simulink model "piddiscreto"  (Simulink 4.00)
settings: Solver=ode45  StartTime=0.0  StopTime=10.0  RelTol=1e-3
settings Model: LastModifiedBy=Gui

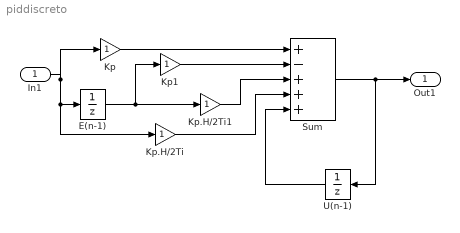
== system piddiscreto ==
  In1 : Inport  Port=1  LatchInput=off
  E(n-1) : UnitDelay  X0=0  SampleTime=0.005
      settings: RTWStateStorageClass=Auto
  Kp : Gain  Gain=1  Multiplication=Element-wise(K.*u)  SaturateOnIntegerOverflow=on
  Kp.H/2Ti : Gain  Gain=1  Multiplication=Element-wise(K.*u)  SaturateOnIntegerOverflow=on
  Kp.H/2Ti1 : Gain  Gain=1  Multiplication=Element-wise(K.*u)  SaturateOnIntegerOverflow=on
  Kp1 : Gain  Gain=1  Multiplication=Element-wise(K.*u)  SaturateOnIntegerOverflow=on
  Sum : Sum  Inputs=+-+++  SaturateOnIntegerOverflow=on
  U(n-1) : UnitDelay  Orientation=left  X0=0  SampleTime=0.005
      settings: RTWStateStorageClass=Auto
  Out1 : Outport  Port=1
  wires:
  In1/1 -> Kp/1, E(n-1)/1, Kp.H/2Ti/1
  Kp/1 -> Sum/1
  E(n-1)/1 -> Kp1/1, Kp.H/2Ti1/1
  Kp1/1 -> Sum/2
  Sum/1 -> U(n-1)/1, Out1/1
  U(n-1)/1 -> Sum/5
  Kp.H/2Ti/1 -> Sum/4
  Kp.H/2Ti1/1 -> Sum/3
